simulink model "ball_model_xy"  (R2015b)
settings: Solver=ode45  StartTime=0.0  StopTime=30  RelTol=1e-3
undefined symbols (not defined in the file): Outx, Outy, S1
libraries: simulink x4, dspvision x1, visionconversions x1, visionstatistics x1
settings Model: Creator=henry  LastModifiedBy=henry
settings DataIOCC: SaveFormat=Array
settings DebuggingCC: SolverPrmCheckMsg=warning
settings HardwareCC: ProdBitPerPointer=32  ProdLargestAtomicFloat=None  ProdIntDivRoundTo=Undefined  ProdEndianess=Unspecified  ProdWordSize=32  ProdHWDeviceType=32-bit Generic
settings ModelReferenceCC: ModelReferenceMinAlgLoopOccurrences=on
settings GRTTargetCC: GeneratePreprocessorConditionals=Disable all
settings ConfigComp: CovModelRefEnable=Off  CovSFcnEnable=off

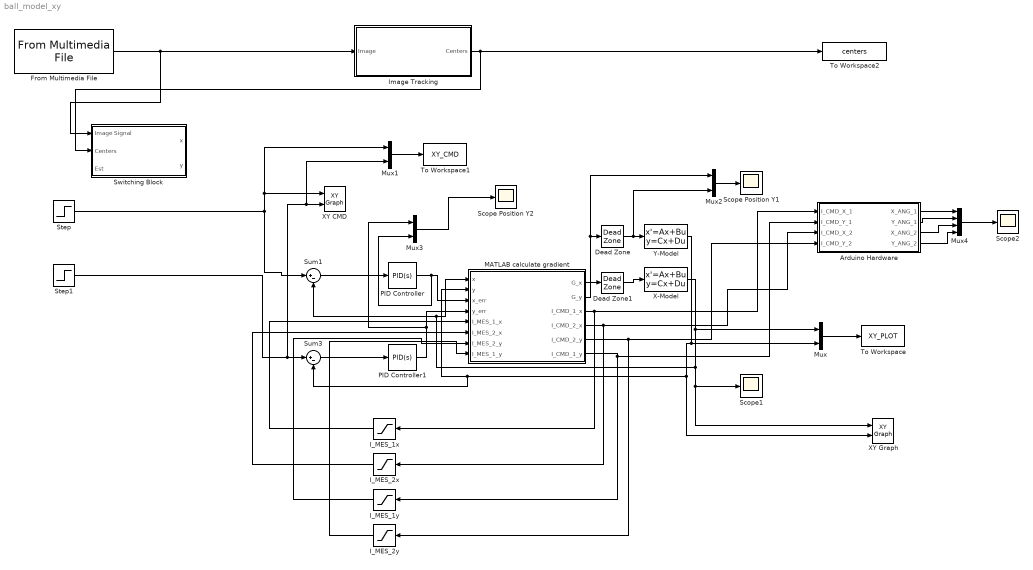
== system ball_model_xy ==
  Arduino Hardware : Subsystem
  Dead Zone : DeadZone  LowerValue=-0.001  UpperValue=0.001  SaturateOnIntegerOverflow=on
  Dead Zone1 : DeadZone  LowerValue=-0.001  UpperValue=0.001  SaturateOnIntegerOverflow=on
  From Multimedia File : dspvision/From Multimedia File  inputFilename=/home/henry/MatLab Homework/UH Special Topics/Gitup/MagneticController/Test Videos/output3.ogg  loop=on  numPlays=inf  outputStreams=Video only  videoDataType=single  audioDataType=int16  inheritSampleTime=on  userDefinedSampleTime=1/30  noAudioOutput=off  isIntensityVideo=off  fourcc=Intensity  colorVideoFormat=One multidimensional signal  outputEOF=off  dataOrg=Column-major  audioFrameSize=1024  computeAudioFrameSize=off  outSamplingMode=Sample based
  I_MES_1x : Saturate  UpperLimit=17  LowerLimit=-17
  I_MES_1y : Saturate  UpperLimit=17  LowerLimit=-17
  I_MES_2x : Saturate  UpperLimit=17  LowerLimit=-17
  I_MES_2y : Saturate  UpperLimit=17  LowerLimit=-17
  Image Tracking : Subsystem
  MATLAB calculate gradient : MATLAB Function  TreatAsAtomicUnit=on
  Mux{,1..3} (4 alike) : Mux  Inputs=2
  Mux4 : Mux
  PID Controller : simulink/Continuous/PID Controller  Controller=PID  TimeDomain=Continuous-time  SampleTime=-1  IntegratorMethod=Forward Euler  FilterMethod=Forward Euler  Form=Parallel  UseFilter=on  ControllerParametersSource=internal  P=1720.64282364148  I=56.1763842699307  D=3243.66405815215  N=8.48230599431706  InitialConditionSource=internal  InitialConditionForIntegrator=0  InitialConditionForFilter=0  ExternalReset=none  LimitOutput=off  UpperSaturationLimit=1  LowerSaturationLimit=-1  LinearizeAsGain=on  AntiWindupMode=back-calculation  Kb=1  TrackingMode=off  Kt=1  PParamMin=[]  PParamMax=[]  IParamMin=[]  IParamMax=[]  DParamMin=[]  DParamMax=[]  NParamMin=[]  NParamMax=[]  KbParamMin=[]  KbParamMax=[]  KtParamMin=[]  KtParamMax=[]  POutMin=[]  POutMax=[]  IOutMin=[]  IOutMax=[]  DOutMin=[]  DOutMax=[]  NOutMin=[]  NOutMax=[]  KbOutMin=[]  KbOutMax=[]  KtOutMin=[]  KtOutMax=[]  IntegratorOutMin=[]  IntegratorOutMax=[]  FilterOutMin=[]  FilterOutMax=[]  SumOutMin=[]  SumOutMax=[]  SumI1OutMin=[]  SumI1OutMax=[]  SumI2OutMin=[]  SumI2OutMax=[]  SumI3OutMin=[]  SumI3OutMax=[]  SumDOutMin=[]  SumDOutMax=[]  SaturationOutMin=[]  SaturationOutMax=[]  IntegratorContinuousStateAttributes=''  IntegratorStateMustResolveToSignalObject=off  IntegratorRTWStateStorageClass=Auto  FilterContinuousStateAttributes=''  FilterStateMustResolveToSignalObject=off  FilterRTWStateStorageClass=Auto  DifferentiatorICPrevScaledInput=0  DifferentiatorOutMin=[]  DifferentiatorOutMax=[]
  PID Controller1 : simulink/Continuous/PID Controller  Controller=PID  TimeDomain=Continuous-time  SampleTime=-1  IntegratorMethod=Forward Euler  FilterMethod=Forward Euler  Form=Parallel  UseFilter=on  ControllerParametersSource=internal  P=44.5562972680473  I=0.115171327894322  D=183.468839848629  N=0.513781942130724  InitialConditionSource=internal  InitialConditionForIntegrator=0  InitialConditionForFilter=0  ExternalReset=none  LimitOutput=off  UpperSaturationLimit=1  LowerSaturationLimit=-1  LinearizeAsGain=on  AntiWindupMode=back-calculation  Kb=1  TrackingMode=off  Kt=1  PParamMin=[]  PParamMax=[]  IParamMin=[]  IParamMax=[]  DParamMin=[]  DParamMax=[]  NParamMin=[]  NParamMax=[]  KbParamMin=[]  KbParamMax=[]  KtParamMin=[]  KtParamMax=[]  POutMin=[]  POutMax=[]  IOutMin=[]  IOutMax=[]  DOutMin=[]  DOutMax=[]  NOutMin=[]  NOutMax=[]  KbOutMin=[]  KbOutMax=[]  KtOutMin=[]  KtOutMax=[]  IntegratorOutMin=[]  IntegratorOutMax=[]  FilterOutMin=[]  FilterOutMax=[]  SumOutMin=[]  SumOutMax=[]  SumI1OutMin=[]  SumI1OutMax=[]  SumI2OutMin=[]  SumI2OutMax=[]  SumI3OutMin=[]  SumI3OutMax=[]  SumDOutMin=[]  SumDOutMax=[]  SaturationOutMin=[]  SaturationOutMax=[]  IntegratorContinuousStateAttributes=''  IntegratorStateMustResolveToSignalObject=off  IntegratorRTWStateStorageClass=Auto  FilterContinuousStateAttributes=''  FilterStateMustResolveToSignalObject=off  FilterRTWStateStorageClass=Auto  DifferentiatorICPrevScaledInput=0  DifferentiatorOutMin=[]  DifferentiatorOutMax=[]
  Scope Position Y1 : Scope
  Scope Position Y2 : Scope
  Scope1 : Scope
  Scope2 : Scope
  Step : Step  SampleTime=0
  Step1 : Step  SampleTime=0
  Sum1 : Sum  Inputs=|+-
  Sum3 : Sum  Inputs=|+-
  Switching Block : Subsystem
  To Workspace : ToWorkspace  VariableName=XY_PLOT  SampleTime=-1
  To Workspace1 : ToWorkspace  VariableName=XY_CMD  SampleTime=-1
  To Workspace2 : ToWorkspace  VariableName=centers  SampleTime=-1
  X-Model : StateSpace  A=[0 1;0 S1]  B=[0;1]  C=[1 0]  D=0  X0=[Outx 0]
  XY CMD : simulink/Sinks/XY Graph  xmin=-0.2  xmax=0.2  ymin=-0.2  ymax=0.2  st=-1
  XY Graph : simulink/Sinks/XY Graph  xmin=-0.2  xmax=0.2  ymin=-0.2  ymax=0.2  st=-1
  Y-Model : StateSpace  A=[0 1;0 S1]  B=[0;1]  C=[1 0]  D=0  X0=[Outy 0]
  wires:
  X-Model/1 -> MATLAB calculate gradient/1(x), Sum1/2, XY Graph/1, Scope1/1, Mux/1
  PID Controller/1 -> Mux3/2, MATLAB calculate gradient/3(x_err)
  Mux/1 -> To Workspace/1
  Y-Model/1 -> MATLAB calculate gradient/2(y), Sum3/2, XY Graph/2, Mux/2
  Sum1/1 -> PID Controller/1
  Sum3/1 -> PID Controller1/1
  PID Controller1/1 -> Mux3/1, MATLAB calculate gradient/4(y_err)
  I_MES_1x/1 -> MATLAB calculate gradient/5(I_MES_1_x)
  I_MES_2x/1 -> MATLAB calculate gradient/6(I_MES_2_x)
  I_MES_1y/1 -> MATLAB calculate gradient/7(I_MES_2_y)
  I_MES_2y/1 -> MATLAB calculate gradient/8(I_MES_1_y)
  MATLAB calculate gradient/3(I_CMD_1_x) -> Arduino Hardware/1(I_CMD_X_1), I_MES_1x/1
  MATLAB calculate gradient/4(I_CMD_2_x) -> Arduino Hardware/3(I_CMD_X_2), I_MES_2x/1
  MATLAB calculate gradient/6(I_CMD_1_y) -> Arduino Hardware/2(I_CMD_Y_1), I_MES_1y/1
  MATLAB calculate gradient/5(I_CMD_2_y) -> Arduino Hardware/4(I_CMD_Y_2), I_MES_2y/1
  Mux1/1 -> To Workspace1/1
  Mux2/1 -> Scope Position Y1/1
  MATLAB calculate gradient/2(G_y) -> Dead Zone/1, Mux2/1
  Dead Zone/1 -> Mux2/2, Y-Model/1
  MATLAB calculate gradient/1(G_x) -> Dead Zone1/1
  Dead Zone1/1 -> X-Model/1
  Mux3/1 -> Scope Position Y2/1
  Step/1 -> Sum1/1, Mux1/1, XY CMD/1
  Step1/1 -> Mux1/2, XY CMD/2, Sum3/1
  Arduino Hardware/1(X_ANG_1) -> Mux4/1
  Arduino Hardware/2(Y_ANG_1) -> Mux4/2
  Mux4/1 -> Scope2/1
  Arduino Hardware/3(X_ANG_2) -> Mux4/3
  Arduino Hardware/4(Y_ANG_2) -> Mux4/4
  From Multimedia File/1 -> Switching Block/1(Image Signal), Image Tracking/1(Image)
  Image Tracking/1(Centers) -> To Workspace2/1, Switching Block/2(Centers)

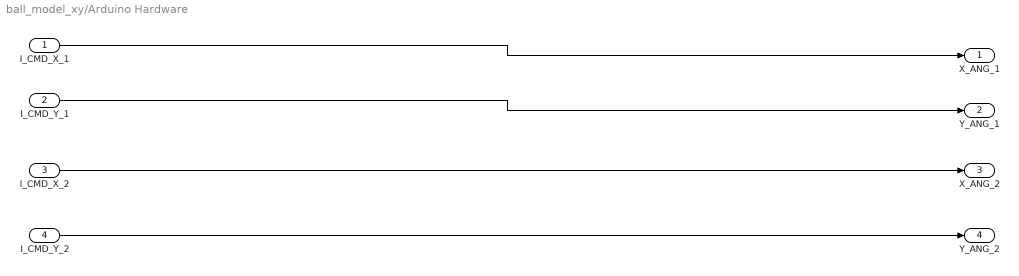
== system ball_model_xy/Arduino Hardware ==
  I_CMD_X_1 : Inport
  I_CMD_Y_1 : Inport  Port=2
  I_CMD_X_2 : Inport  Port=3
  I_CMD_Y_2 : Inport  Port=4
  X_ANG_1 : Outport
  Y_ANG_1 : Outport  Port=2
  X_ANG_2 : Outport  Port=3
  Y_ANG_2 : Outport  Port=4
  wires:
  I_CMD_X_1/1 -> X_ANG_1/1
  I_CMD_Y_1/1 -> Y_ANG_1/1
  I_CMD_X_2/1 -> X_ANG_2/1
  I_CMD_Y_2/1 -> Y_ANG_2/1

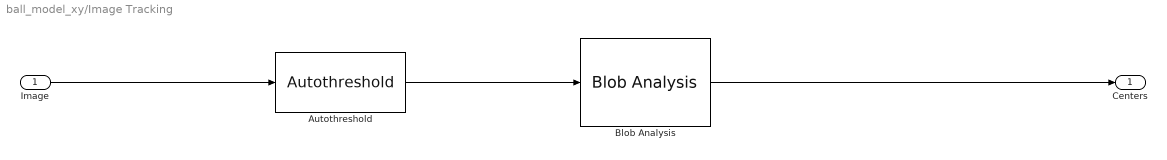
== system ball_model_xy/Image Tracking ==
  Image : Inport
  Autothreshold : visionconversions/Autothreshold  operator=>  threshOut=off  effMetricOut=off  userDefinedRange=off  umin=0  umax=255  outOfRngOpt=Warn and saturate  scaleThreshold=off  scaleFactor=1  P1Mode=Specify word length  P1WordLength=32  P1FracLength=30  P2Mode=Specify word length  P2WordLength=32  P2FracLength=22  P3Mode=Specify word length  P3WordLength=32  P3FracLength=14  P4Mode=Binary point scaling  P4WordLength=32  P4FracLength=15  Q1Mode=Specify word length  Q1WordLength=32  Q1FracLength=16  EMMode=Specify word length  EMWordLength=16  EMFracLength=14  roundingMode=Floor  overflowMode=off
  Blob Analysis : visionstatistics/Blob Analysis  Tag=vipblks_row_conv  area=off  centroid=on  bBox=off  majorAxis=off  minorAxis=off  angle=off  eccentricity=off  equivDiameterSq=off  extent=off  perimeter=off  maxBlobs=1  warnIfNumBlobsExceeded=off  isCount=off  useMinArea=on  minArea=2000  useMaxArea=on  maxArea=3000  excludeBorderBlob=on  outDT=double  isOutVarDim=off  isFill=off  fillValues=-1  conn=8  isLabel=off  outputMode=Binary point scaling  outputWordLength=32  outputFracLength=16  firstCoeffMode=Binary point scaling  firstCoeffWordLength=16  firstCoeffFracLength=14  secondCoeffMode=Binary point scaling  secondCoeffWordLength=32  secondCoeffFracLength=16  accumMode=Binary point scaling  accumWordLength=32  accumFracLength=0  prodOutputMode=Binary point scaling  prodOutputWordLength=32  prodOutputFracLength=16  roundingMode=Floor  overflowMode=off
  Centers : Outport
  wires:
  Image/1 -> Autothreshold/1
  Autothreshold/1 -> Blob Analysis/1
  Blob Analysis/1 -> Centers/1

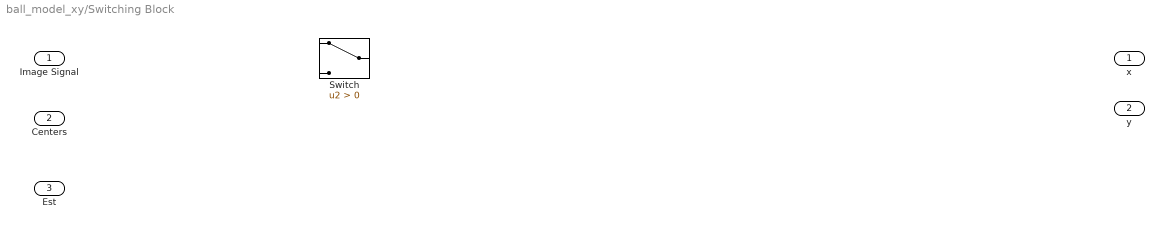
== system ball_model_xy/Switching Block ==
  Image Signal : Inport
  Centers : Inport  Port=2
  Est : Inport  Port=3
  Switch : Switch  Criteria=u2 > Threshold
  x : Outport
  y : Outport  Port=2

== matlab function ball_model_xy/MATLAB calculate gradient ==
  data: x input; y input; x_err input; y_err input; G_x output; G_y output; I_MES_1_x input; I_CMD_1_x output; I_MES_2_x input; I_CMD_2_x output; I_MES_2_y input; I_MES_1_y input; I_CMD_2_y output; I_CMD_1_y output
function [G_x,G_y,I_CMD_1_x,I_CMD_2_x,I_CMD_2_y,I_CMD_1_y] = BGrad(x,y,x_err,y_err,I_MES_1_x,I_MES_2_x,I_MES_2_y,I_MES_1_y)
%#codegen
%Model of Magnetix Fields
N = 510; %number of coils
M=1;
W = 0.001;
u_o =(4*3.14*10^(-7));
uk = 0.47;
FN = 9.81*W
FF = (uk*FN)/W;
%I_1 = 17 %Max current through coil in A
%I_2 = 17
R =0.08; %radius of coil in meters
R_1=0.01;
%s = linspace(0,10)
%b_z=0:99
%b_z_2=0:99
%b_z_total=0:99
%z = 0;
%z_2 = 0.1;

%for k=1:100

V = (4/3)*(3.14)*(R_1^3);
x=x+0.0001;
y=y+0.0001;

x1=x;
y1=y;

x2=0.1-x;
y2=0.1-y;
%z_2 = z_2-0.001
%b_x = (u_o*N*I_MES*(R^2))/((2*((R^2)+(x^2)))^1.5);
%b_z_2(k) = (u_o*N*I_1*(R^2))/((2*((R^2)+(z_2^2)))^1.5)
%b_z_total(k) = b_z(k)+b_z_2(k)
%db_z = (-3*u_o*N*I*(R^2)*z)/(((R^2)+(z^2))^2.5)\

%db_z_1(k) = (u_o*N*I_1*(R^2)*((-3*z)))/(2*(((R^2)+(z^2))^(2.5)));

db_x_1 = M*V*(u_o*N*I_MES_1_x*(R^2)*((-3*x1)))/(2*((R^2)+(x1^2))^(2.5));
db_y_1 = M*V*(u_o*N*I_MES_1_y*(R^2)*((-3*y1)))/(2*((R^2)+(y1^2))^(2.5));

db_x_2 = M*V*(u_o*N*I_MES_2_x*(R^2)*((-3*x2)))/(2*((R^2)+(x2^2))^(2.5));
db_y_2 = M*V*(u_o*N*I_MES_2_y*(R^2)*((-3*y2)))/(2*((R^2)+(y2^2))^(2.5));

%G_x = ((db_x_1+db_x_2)/W)*x_err;
%G_y = ((db_y_1+db_y_2)/W)*y_err;

G_x = ((db_x_1+db_x_2)/W);
G_y = ((db_y_1+db_y_2)/W);

%I_CMD_1 = x_err*(db_x_1*((R^2)+(x1^2))^(2.5))/(-3*x1*u_o*N*(R^2));
%I_CMD_2 = y_err*(db_x_2*((R^2)+(x2^2))^(2.5))/(-3*x2*u_o*N*(R^2));

I_CMD_1_x = x_err*(-17);
I_CMD_2_x = x_err*(-17);
I_CMD_1_y = y_err*(-17);
I_CMD_2_y = y_err*(-17);


%I_CMD = -5*I_set;

%I_CMD = x_err*17
%db_z_2(k) = (u_o*N*I_2*(R^2)*((-3*z_2)))/(((R^2)+(z_2^2))^(2.5))
%db_z_total(k) = db_z_1(k)+db_z_2(k)
%end
%plot(s,b_z,s,b_z_2,s,b_z_total)
%plot(s,db_z_1,s,db_z_2,s,db_z_total)
%ylabel('T - Telsa') 
%xlabel('distance - cm')
%I_CMD = 0.01;
